simulink model "CelsiusConverter_JamesWilkinson"  (R2025a)
settings: Solver=VariableStepAuto  StartTime=0.0  StopTime=10.0  RelTol=1e-3
settings Model: Creator=james  LastModifiedBy=james

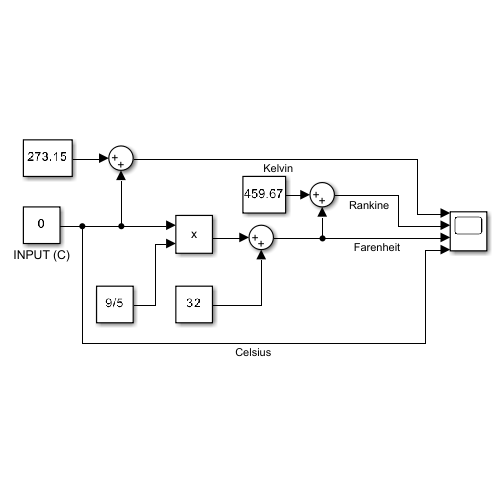
[thumbnail: Simulink's stored preview of the top-level diagram]
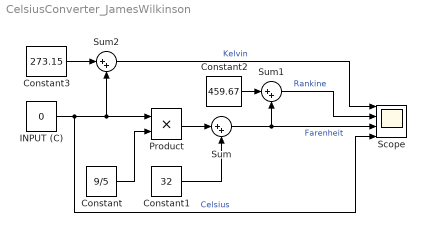
== system CelsiusConverter_JamesWilkinson ==
  Constant : Constant  Value=9/5
  Constant1 : Constant  Value=32
  Constant2 : Constant  Value=459.67
  Constant3 : Constant  Value=273.15
  INPUT (C) : Constant  Value=0
  Product : Product
  Scope : Scope  NumInputPorts=4
      settings: ActiveDisplayYMinimum=-61.458749999999988  ActiveDisplayYMaximum=553.12875  YLabel=Temp (in respective units)
  Sum : Sum  Inputs=|++
  Sum1 : Sum  Inputs=|++
  Sum2 : Sum  Inputs=|++
  wires:
  INPUT (C)/1 -> Sum2/2, Product/1, Scope/4  "Celsius"
  Constant/1 -> Product/2
  Product/1 -> Sum/1
  Constant1/1 -> Sum/2
  Sum/1 -> Scope/3, Sum1/2  "Farenheit"
  Constant3/1 -> Sum2/1
  Constant2/1 -> Sum1/1
  Sum2/1 -> Scope/1  "Kelvin"
  Sum1/1 -> Scope/2  "Rankine"
